simulink model "H175_Stage_01_Anode_Cathode"  (R2023a)
settings: Solver=VariableStepAuto  StartTime=0.0  StopTime=500  RelTol=1e-3
values from neighbouring files (symbols this model uses):
  anode_tube_D = 0.01    [All_Properties.mat]    (also in anode_subsystem_parameters.m; environment_parameters.m)
  D = 0.01    [All_Properties.mat]    (also in anode_subsystem_parameters.m)
  densityHydrogen = 0.0899    [All_Properties.mat]    (also in Valve_Init.m; anode_subsystem_parameters.m)
  Fischer_EMTC120K_supplier_mdot_TLU = [33.385172 57.11265182 82.35238332 173.9183787 230.2050798 50.1655574 86.1774137 122.96585 210.0188714 258.8737112 70.20710678 115.3896052 ... (25 elements, 5x5)]    [All_Properties.mat]    (also in cathode_subsystem_parameters.m = [33.385172 50.1655574 70.20710678 87.4902972 105.3161257)
  Fischer_EMTC120K_supplier_pr_TLU = [2.452176848 3.067593046 4.01020547 5.11549365 6.10066015 2.450765612 3.07166407 4.0616557 5.112468546 6.108742034 2.432340262 3.033516574 ... (25 elements, 5x5)]    [All_Properties.mat]    (also in cathode_subsystem_parameters.m = [2.452176848 2.450765612 2.432340262 2.407245766 2.37067916)
  Kv_VL6112 = 0.8    [All_Properties.mat]    (also in anode_subsystem_parameters.m)
  N2_T = [-56.55 -50 -40 -30 -20 -10 -5 -4 -3 -2 -1 0 ... (52 elements, 1x52)]    [All_Properties.mat]    (also in anode_subsystem_parameters.m = [-56.55 -50 -40 -30 -20 -10 -5 -4 -3 -2 -1 0 1 2 3 4 5 10 20; environment_parameters.m = [-56.55, -50:10:-10, -5:1:5, 10:10:350]; stack_model_harness_parameters.m = [-56.55, -50:10:-10, -5:1:5, 10:10:350])
  p_range = 0.005    [All_Properties.mat]    (also in anode_subsystem_parameters.m)
  r_max = 0.2    [All_Properties.mat]    (also in anode_subsystem_parameters.m)
  r_min = 0.0001    [All_Properties.mat]    (also in anode_subsystem_parameters.m)
  responseTimeValve = 0.013    [All_Properties.mat]    (also in anode_subsystem_parameters.m)
undefined symbols (not defined in the file or in its folder): sigbuilder_block
libraries: fl_lib x168, nesl_utility x116, SimscapeFluids_lib x8, slpidlib x5, simulink x1
(part 3 of 8)

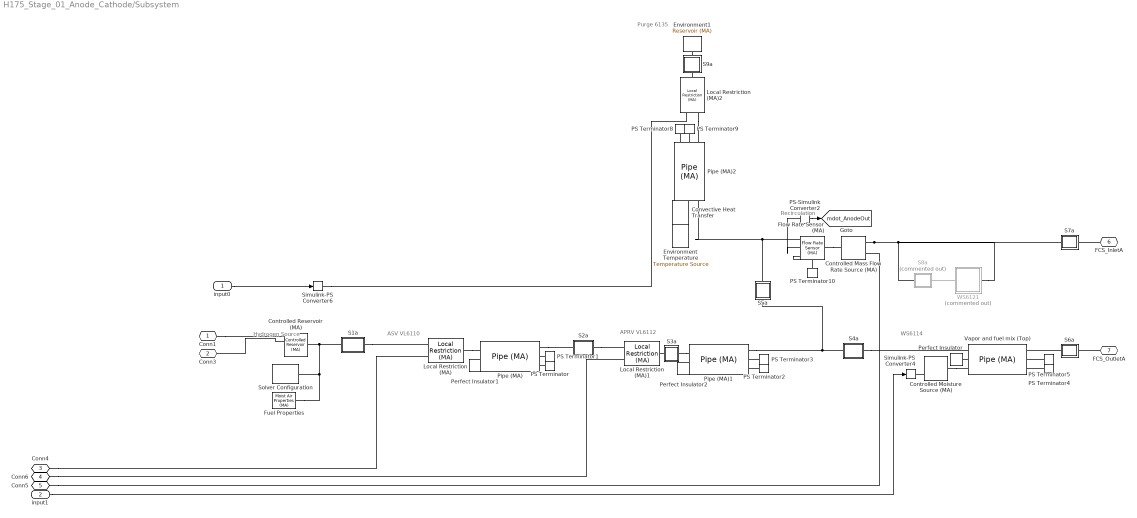
== system H175_Stage_01_Anode_Cathode/Subsystem ==
  note: Purge 6135
  note: Recirculation
  note: WS6114
  note: APRV VL6112
  note: ASV VL6110
  note: Hydrogen Source
  input0 : Inport
  input1 : Inport  Port=2
  " WS6121" : Subsystem  Tag=PublishSubsystem  Commented=on
  Controlled Mass Flow Rate Source (MA) : fl_lib/Moist Air/Sources/Controlled Mass Flow Rate Source (MA)  power_spec=foundation.enum.power_spec.isentropic  area_A=pi*anode_tube_D^2/4 m^2  area_B=pi*anode_tube_D^2/4 m^2
      settings: InternalSimscapePortConfiguration="{\"Bottom\":[],\"Left\":[{\"id\":\"A\",\"label\":\"A\",\"type\":\"foundation.moist_air.moist_air\"},{\"id\":\"M\",\"label\":\"M\",\"type\":\"input\"}],\"Right\":[{\"id\":\"B\",\"label\":\"B\",\"type\":\"foundation.moist_air.moist_air\"}],\"Top\":[]}"
  Controlled Moisture Source (MA) : fl_lib/Moist Air/Sources/Moisture & Trace Gas Sources/Controlled Moisture Source (MA)  moisture_source_spec=foundation.enum.moisture_source_spec.liquid  Phi_S_specify=off  Phi_S_priority=None  Phi_S=0 kW  Phi_S_nominal_specify=off  Phi_S_nominal_unit=kW  Phi_S_nominal_value=1  mdot_w_S_specify=off  mdot_w_S_priority=None  mdot_w_S=0 kg/s  mdot_w_S_nominal_specify=off  mdot_w_S_nominal_unit=kg/s  mdot_w_S_nominal_value=1
      settings: InternalSimscapePortConfiguration="{\"Bottom\":[],\"Left\":[{\"id\":\"S\",\"label\":\"S\",\"type\":\"foundation.moist_air.moist_air_source\"}],\"Right\":[{\"id\":\"M\",\"label\":\"M\",\"type\":\"input\"},{\"id\":\"T\",\"label\":\"T\",\"type\":\"input\"}],\"Top\":[]}"
  Controlled Reservoir (MA) : fl_lib/Moist Air/Elements/Controlled Reservoir (MA)  moisture_spec=foundation.enum.moistureSpec.RelativeHumidity  trace_gas_spec=foundation.enum.trace_gas_spec.mass_fraction  RH_ws=1  area_A=0.01 m^2  input_error_spec=foundation.enum.input_range_error.warn
      settings: InternalSimscapePortConfiguration="{\"Bottom\":[],\"Left\":[{\"id\":\"A\",\"label\":\"A\",\"type\":\"foundation.moist_air.moist_air\"}],\"Right\":[{\"id\":\"T\",\"label\":\"T\",\"type\":\"input\"},{\"id\":\"P\",\"label\":\"P\",\"type\":\"input\"},{\"id\":\"W\",\"label\":\"W\",\"type\":\"input\"},{\"id\":\"G\",\"label\":\"G\",\"type\":\"input\"}],\"Top\":[]}"
  Convective Heat Transfer : fl_lib/Thermal/Thermal Elements/Convective Heat Transfer  thermal_type=foundation.enum.constant_variable.constant  area=pi*anode_tube_D*1 m^2  heat_tr_coeff=20 W/(m^2 * K)  min_heat_tr_coeff=1e-3 W/(K*m^2)  T_specify=off  T_priority=None  T=0 K  T_nominal_specify=off  T_nominal_unit=K  T_nominal_value=1  Q_specify=off  Q_priority=None  Q=0 W  Q_nominal_specify=off  Q_nominal_unit=W  Q_nominal_value=1
  Environment Temperature : fl_lib/Thermal/Thermal Sources/Temperature Source  temperature=env_T degC
  Environment1 : fl_lib/Moist Air/Elements/Reservoir (MA)  pressure_spec=foundation.enum.pressure_spec.atmospheric  reservoir_pressure=0.101325 MPa  temperature_spec=foundation.enum.temperature_spec.atmospheric  reservoir_temperature=293.15 K  moisture_spec=foundation.enum.moistureSpec.RelativeHumidity  reservoir_RH=0.5  reservoir_x_w=0.01  reservoir_y_w=0.01  reservoir_HR=0.01  reservoir_Tw=287 K  trace_gas_spec=foundation.enum.trace_gas_spec.mass_fraction  reservoir_x_g=0.001  reservoir_y_g=0.001  RH_ws=1  area_A=0.01 m^2
  Flow Rate Sensor (MA) : fl_lib/Moist Air/Sensors/Flow Rate Sensor (MA)  mass_flow_measure=true  volumetric_flow_measure=false  volumetric_flow_conditions=foundation.enum.volumetric_flow_conditions.actual  p_std=0.101325 MPa  T_std=20 degC  RH_std=0.65  energy_flow_measure=true  vapor_flow_measure=false  gas_flow_measure=false
      settings: InternalSimscapePortConfiguration="{\"Bottom\":[{\"id\":\"PHI\",\"label\":\"φ\",\"type\":\"output\"}],\"Left\":[{\"id\":\"A\",\"label\":\"A\",\"type\":\"foundation.moist_air.moist_air\"}],\"Right\":[{\"id\":\"B\",\"label\":\"B\",\"type\":\"foundation.moist_air.moist_air\"},{\"id\":\"M\",\"label\":\"M\",\"type\":\"output\"}],\"Top\":[]}"
  Fuel Properties : fl_lib/Moist Air/Utilities/Moist Air Properties (MA)  R_a=N2_R J/kg/K  T_TLU=N2_T degC  h_a_TLU=N2_h kJ/kg  mu_a_TLU=N2_mu s*uPa  k_a_TLU=N2_k mW/m/K  p_min=1 kPa  p_max=inf MPa  T_min=min(N2_T) degC  T_max=max(N2_T) degC  properties_range_check=simscape.enum.assert.action.error  p_atm=0.101325 MPa  T_atm=20 degC  R_w=461.523 J/kg/K  p_ws_TLU=[1.71168953425982e-06; 3.93770601979424e-06; 1.28411717710344e-05; 3.80051394873809e-05; .00010323902900209; .000259873810798063; .000401741022116384; .000437454836117844; .000476040820618202; .000517704666185737; .000562664883741207; .000611212677444345; .000657088049117899; .000705987905898279; .000758082381149132; .000813549384183233; .000872574861129522; .00122818386934022; .0023392147667769; .00424668834054807; .00738442748706953; .0123512704340234; .0199458019246787; .0312006356960619; .0474147199263783; .0701823607447713; .10141797792131; .143375967241115; .198665399739302; .270259606559999; .361500961984849; .476101381081492; .618139196722055; .792053183687694; 1.0026345688121; 1.25501792086105; 1.55467186826983; 1.90739066433297; 2.31928772772542; 2.79679245576864; 3.34665187151016; 3.97593907083533; 4.69207105435535; 5.5028394740883; 6.41645928168037; 7.4416425436169; 8.58770832955728; 9.86474556030261; 11.2838558865497; 12.8575218898034; 14.6001810568052; 16.5291642526045] MPa  h_w_vap_TLU=[2836.88241275372; 2837.81392500514; 2838.63937175807; 2838.7309929628; 2838.06905313927; 2836.62597341095; 2835.60023952573; 2835.37006381376; 2835.13143158077; 2834.88429145066; 2834.62859062897; 2500.93420564316; 2498.55329907119; 2496.17495082036; 2493.79885912205; 2491.42474723191; 2489.05236104642; 2477.20875029194; 2453.54955988604; 2429.83856603313; 2406.00136954922; 2381.97406342174; 2357.69101156389; 2333.08088387814; 2308.06565480412; 2282.56034405021; 2256.47287422313; 2229.70428017508; 2202.14968030993; 2173.69998896199; 2144.24368406447; 2113.66758247452; 2081.85585110571; 2048.68725710494; 2014.03141249899; 1977.7449923284; 1939.66849592886; 1899.62342931686; 1857.40930169838; 1812.79975416601; 1765.53721731251; 1715.32525772152; 1661.81700477787; 1604.59703745016; 1543.1534616334; 1476.83692476464; 1404.80240352424; 1325.92091736114; 1238.61667822208; 1140.5102987018; 1027.62017777647; 892.733785613825] kJ/kg  h_w_TLU=[2396.55944251649; 2408.68643343608; 2427.1988031141; 2445.702165897; 2464.18429108356; 2482.62529466839; 2491.82135326629; 2493.6580151792; 2495.49372578218; 2497.32843835745; 2499.16210446923; 2500.99462758899; 2502.83092214066; 2504.6665223621; 2506.50140563013; 2508.335548891; 2510.16892865793; 2519.32352241995; 2537.56068088674; 2555.67742615292; 2573.6403223998; 2591.4109179101; 2608.9455037701; 2626.19492016262; 2643.10444358428; 2659.61377634497; 2675.58278696023; 2696.1846256545; 2716.49989553741; 2736.6235210957; 2756.61216047011; 2776.50561773853; 2796.33378922508; 2816.11979583049; 2835.88181423877; 2855.63430574511; 2875.38889327595; 2895.15500577172; 2914.94035964689; 2934.75132290228; 2954.59319330244; 2974.47041285505; 2994.38673458964; 3014.34535328009; 3034.34900867103; 3054.40006755764; 3074.50058946898; 3094.65237953784; 3114.85703128106; 3135.11596137801; 3155.43043805905; 3175.80160435813] kJ/kg  mu_w_TLU=[6.81365662228272; 7.04953750742707; 7.40970098298307; 7.76991278093907; 8.13017290129507; 8.49048134405107; 8.67065368632907; 8.70668960445667; 8.74272600580827; 8.77876289038387; 8.81480025818347; 8.85083810920707; 8.88687644345467; 8.92291526092627; 8.95895456162187; 8.99499434554147; 9.03103461268507; 9.21124319676307; 9.57169660671907; 9.93219833907507; 10.2927483938311; 10.6533467709871; 11.0139934705431; 11.3746884924991; 11.7354318368551; 12.0962235036111; 12.4570634927671; 12.8179518043231; 13.1788884382791; 13.5398733946351; 13.9009066733911; 14.2619882745471; 14.6231181981031; 14.9842964440591; 15.3455230124151; 15.7067979031711; 16.0681211163271; 16.4294926518831; 16.7909125098391; 17.1523806901951; 17.5138971929511; 17.8754620181071; 18.2370751656631; 18.5987366356191; 18.9604464279751; 19.3222045427311; 19.6840109798871; 20.0458657394431; 20.4077688213991; 20.7697202257551; 21.1317199525111; 21.4937680016671] s*uPa  k_w_TLU=[11.46288215976; 11.941997488935; 12.676358586935; 13.414208884935; 14.155548382935; 14.900377080935; 15.274099879935; 15.348949115735; 15.423833243535; 15.498752263335; 15.573706175135; 15.648694978935; 15.723718674735; 15.798777262535; 15.873870742335; 15.948999114135; 16.024162377935; 16.400502076935; 17.155798374935; 17.914583872935; 18.676858570935; 19.442622468935; 20.211875566935; 20.984617864935; 21.760849362935; 22.540570060935; 23.323779958935; 24.110479056935; 24.900667354935; 25.694344852935; 26.491511550935; 27.292167448935; 28.096312546935; 28.903946844935; 29.715070342935; 30.529683040935; 31.347784938935; 32.169376036935; 32.994456334935; 33.823025832935; 34.655084530935; 35.490632428935; 36.329669526935; 37.172195824935; 38.018211322935; 38.867716020935; 39.720709918935; 40.577193016935; 41.437165314935; 42.300626812935; 43.167577510935; 44.038017408935] mW/m/K  D_w=25 mm^2/s  trace_gas_model=foundation.enum.trace_gas_model.track_properties  R_g=H2_R J/kg/K  h_g_TLU=H2_h kJ/kg  mu_g_TLU=H2_mu s*uPa  k_g_TLU=H2_k mW/m/K  D_g=H2_D mm^2/s
      settings: AttributesFormatString=|
      | dry air --> N2
      | water vapor --> H2O
      | trace gas --> H2
  Local Restriction (MA) : fl_lib/Moist Air/Elements/Local Restriction (MA)  restriction_type=foundation.enum.restriction_type.variable  restriction_area=0.005 m^2  min_area=0.00001e-6 m^2  max_area=4.75e-6 m^2  area=0.00358 m^2  Cd=0.80  B_lam=0.999
      settings: LogSimulationData=on
  Local Restriction (MA)1 : fl_lib/Moist Air/Elements/Local Restriction (MA)  restriction_type=foundation.enum.restriction_type.variable  restriction_area=0.005 m^2  min_area=0.00001e-6 m^2  max_area=4.75e-6 m^2  area=0.00358 m^2  Cd=0.80  B_lam=0.999
      settings: LogSimulationData=on
  Local Restriction (MA)2 : fl_lib/Moist Air/Elements/Local Restriction (MA)  restriction_type=foundation.enum.restriction_type.variable  restriction_area=0.005 m^2  min_area=0.00001e-6 m^2  max_area=3.2e-6 m^2  area=0.00358 m^2  Cd=0.80  B_lam=0.999
      settings: LogSimulationData=on
  PS Terminator{,1..5,8..10} (9 alike) : fl_lib/Physical Signals/Sinks/PS Terminator
  PS-Simulink Converter2 : nesl_utility/PS-Simulink Converter  PhysicalDomain=network_engine_domain  SubClassName=ps_output  LeftPortType=input  RightPortType=output  PseudoPeriodic=off  Frequencies=[]  VectorFormat=inherit  Unit=inherit  AffineConversion=off
  Perfect Insulator : fl_lib/Thermal/Thermal Elements/Perfect Insulator  T_specify=off  T_priority=None  T=0 K  T_nominal_specify=off  T_nominal_unit=K  T_nominal_value=1
  Perfect Insulator1 : fl_lib/Thermal/Thermal Elements/Perfect Insulator  T_specify=off  T_priority=None  T=0 K  T_nominal_specify=off  T_nominal_unit=K  T_nominal_value=1
  Perfect Insulator2 : fl_lib/Thermal/Thermal Elements/Perfect Insulator  T_specify=off  T_priority=None  T=0 K  T_nominal_specify=off  T_nominal_unit=K  T_nominal_value=1
  Pipe (MA) : fl_lib/Moist Air/Elements/Pipe (MA)  length=1 m  area=pi*anode_tube_D^2/4 m^2  Dh=anode_tube_D m  length_add=0.1 m  roughness=15e-6 m  Re_lam=2000  Re_tur=4000  shape_factor=64  Nu_lam=3.66  wall_condensation=simscape.enum.onoff.off  RH_ws=1  time_constant=1e-3 s  moisture_trace_gas_source=foundation.enum.moisture_trace_gas_source.none  moisture_source_spec=foundation.enum.moisture_source_spec.vapor  moisture_mass_flow=0 kg/s  moisture_temperature_spec=foundation.enum.temperature_spec.atmospheric  moisture_temperature=293.15 K  trace_gas_mass_flow=0 kg/s  trace_gas_temperature_spec=foundation.enum.temperature_spec.atmospheric  trace_gas_temperature=293.15 K  p_I_specify=on  p_I_priority=High  p_I=env_p MPa  p_I_nominal_specify=off  p_I_nominal_unit=MPa  p_I_nominal_value=1  T_I_specify=on  T_I_priority=High  T_I=env_T degC  T_I_nominal_specify=off  T_I_nominal_unit=K  T_I_nominal_value=1  RH_I_specify=off  RH_I_priority=High  RH_I=0  RH_I_nominal_specify=off  RH_I_nominal_unit=1  RH_I_nominal_value=1  x_w_I_specify=off  x_w_I_priority=None  x_w_I=0  x_w_I_nominal_specify=off  x_w_I_nominal_unit=1  x_w_I_nominal_value=1  y_w_I_specify=off  y_w_I_priority=None  y_w_I=0  y_w_I_nominal_specify=off  y_w_I_nominal_unit=1  y_w_I_nominal_value=1  HR_I_specify=off  HR_I_priority=None  HR_I=0  HR_I_nominal_specify=off  HR_I_nominal_unit=1  HR_I_nominal_value=1  x_g_I_specify=on  x_g_I_priority=None  x_g_I=0  x_g_I_nominal_specify=off  x_g_I_nominal_unit=1  x_g_I_nominal_value=1  y_g_I_specify=on  y_g_I_priority=High  y_g_I=tank_yH2  y_g_I_nominal_specify=off  y_g_I_nominal_unit=1  y_g_I_nominal_value=1
  Pipe (MA)1 : fl_lib/Moist Air/Elements/Pipe (MA)  length=1 m  area=pi*anode_tube_D^2/4 m^2  Dh=anode_tube_D m  length_add=0.1 m  roughness=15e-6 m  Re_lam=2000  Re_tur=4000  shape_factor=64  Nu_lam=3.66  wall_condensation=simscape.enum.onoff.off  RH_ws=1  time_constant=1e-3 s  moisture_trace_gas_source=foundation.enum.moisture_trace_gas_source.none  moisture_source_spec=foundation.enum.moisture_source_spec.vapor  moisture_mass_flow=0 kg/s  moisture_temperature_spec=foundation.enum.temperature_spec.atmospheric  moisture_temperature=293.15 K  trace_gas_mass_flow=0 kg/s  trace_gas_temperature_spec=foundation.enum.temperature_spec.atmospheric  trace_gas_temperature=293.15 K  p_I_specify=on  p_I_priority=High  p_I=env_p MPa  p_I_nominal_specify=off  p_I_nominal_unit=MPa  p_I_nominal_value=1  T_I_specify=on  T_I_priority=High  T_I=env_T degC  T_I_nominal_specify=off  T_I_nominal_unit=K  T_I_nominal_value=1  RH_I_specify=off  RH_I_priority=High  RH_I=0  RH_I_nominal_specify=off  RH_I_nominal_unit=1  RH_I_nominal_value=1  x_w_I_specify=off  x_w_I_priority=None  x_w_I=0  x_w_I_nominal_specify=off  x_w_I_nominal_unit=1  x_w_I_nominal_value=1  y_w_I_specify=off  y_w_I_priority=None  y_w_I=0  y_w_I_nominal_specify=off  y_w_I_nominal_unit=1  y_w_I_nominal_value=1  HR_I_specify=off  HR_I_priority=None  HR_I=0  HR_I_nominal_specify=off  HR_I_nominal_unit=1  HR_I_nominal_value=1  x_g_I_specify=on  x_g_I_priority=None  x_g_I=0  x_g_I_nominal_specify=off  x_g_I_nominal_unit=1  x_g_I_nominal_value=1  y_g_I_specify=on  y_g_I_priority=High  y_g_I=tank_yH2  y_g_I_nominal_specify=off  y_g_I_nominal_unit=1  y_g_I_nominal_value=1
  Pipe (MA)2 : fl_lib/Moist Air/Elements/Pipe (MA)  length=1 m  area=pi*anode_tube_D^2/4 m^2  Dh=anode_tube_D m  length_add=0.1 m  roughness=15e-6 m  Re_lam=2000  Re_tur=4000  shape_factor=64  Nu_lam=3.66  wall_condensation=simscape.enum.onoff.off  RH_ws=1  time_constant=1e-3 s  moisture_trace_gas_source=foundation.enum.moisture_trace_gas_source.none  moisture_source_spec=foundation.enum.moisture_source_spec.vapor  moisture_mass_flow=0 kg/s  moisture_temperature_spec=foundation.enum.temperature_spec.atmospheric  moisture_temperature=293.15 K  trace_gas_mass_flow=0 kg/s  trace_gas_temperature_spec=foundation.enum.temperature_spec.atmospheric  trace_gas_temperature=293.15 K  p_I_specify=on  p_I_priority=High  p_I=env_p MPa  p_I_nominal_specify=off  p_I_nominal_unit=MPa  p_I_nominal_value=1  T_I_specify=on  T_I_priority=High  T_I=env_T degC  T_I_nominal_specify=off  T_I_nominal_unit=K  T_I_nominal_value=1  RH_I_specify=off  RH_I_priority=High  RH_I=0  RH_I_nominal_specify=off  RH_I_nominal_unit=1  RH_I_nominal_value=1  x_w_I_specify=off  x_w_I_priority=None  x_w_I=0  x_w_I_nominal_specify=off  x_w_I_nominal_unit=1  x_w_I_nominal_value=1  y_w_I_specify=off  y_w_I_priority=None  y_w_I=0  y_w_I_nominal_specify=off  y_w_I_nominal_unit=1  y_w_I_nominal_value=1  HR_I_specify=off  HR_I_priority=None  HR_I=0  HR_I_nominal_specify=off  HR_I_nominal_unit=1  HR_I_nominal_value=1  x_g_I_specify=on  x_g_I_priority=None  x_g_I=0  x_g_I_nominal_specify=off  x_g_I_nominal_unit=1  x_g_I_nominal_value=1  y_g_I_specify=on  y_g_I_priority=High  y_g_I=tank_yH2  y_g_I_nominal_specify=off  y_g_I_nominal_unit=1  y_g_I_nominal_value=1
  S1a : Subsystem
  S2a : Subsystem
  S3a : Subsystem
  S4a : Subsystem
  S5a : Subsystem
  S6a : Subsystem
  S7a : Subsystem  Tag=PublishSubsystem
  S8a : Subsystem  Tag=PublishSubsystem  Commented=on
  S9a : Subsystem
  Simulink-PS Converter4 : nesl_utility/Simulink-PS Converter  PhysicalDomain=network_engine_domain  SubClassName=ps_input  LeftPortType=input  RightPortType=output  PseudoPeriodic=off  Frequencies=[]  NoiseDistribution=none  NoiseParameters=[]  Unit=1  AffineConversion=off  FilteringAndDerivatives=provide  SimscapeFilterOrder=1  InputFilterTimeConstant=0.001  UdotUserProvided=0
  Simulink-PS Converter6 : nesl_utility/Simulink-PS Converter  PhysicalDomain=network_engine_domain  SubClassName=ps_input  LeftPortType=input  RightPortType=output  PseudoPeriodic=off  Frequencies=[]  NoiseDistribution=none  NoiseParameters=[]  Unit=1  AffineConversion=off  FilteringAndDerivatives=provide  SimscapeFilterOrder=1  InputFilterTimeConstant=0.001  UdotUserProvided=0
  Solver Configuration : nesl_utility/Solver Configuration  PhysicalDomain=network_engine_domain  SubClassName=solver  LeftPortType=input  RightPortType=generic  Tones=[]  Harmonics=[]  SimulateNoise=off  Profile=off  UseLocalSampling=off  EnableSwitchedLinearOptims=on  FrequencyDomain=off  UseCCode=off  RelTol=0.001  AbsTol=0.001  MinStep=1e-09  ToWorkspace=off  RevertToSquareIcSolve=off  NumHomotopyIterations=100  PhasorMode=off  PhasorModeNumHarmonics=1  ConsistencySolver=NEWTON_XTOL_AFTER_FTOL  IndexReductionMethod=DerivativeReplacement  DoDC=off  ResidualTolerance=1e-09  ConsistencyTolSource=GLOBAL  ConsistencyAbsTol=0.001  ConsistencyRelTol=0.001  ConsistencyTolFactor=0.001  UseLocalSolver=off  LocalSolverChoice=NE_BACKWARD_EULER_ADVANCER  ResolveIndetEquations=on  FunctionEvalNumThread=1  LocalSolverSampleTime=0.001  DoFixedCost=off  MaxNonlinIter=3  MaxModeIter=2  ComputeImpulses=off  ImpulseIterations=2  LinearAlgebra=auto  LinearAlgebraNumThread=0  EquationFormulation=NE_TIME_EF  DelaysMemoryBudget=1024  AutomaticFiltering=on  FilteringTimeConstant=0.001  PartitionStorageMethod=AS_NEEDED  PartitionMemoryBudget=1024  PartitionMethod=ROBUST
  Vapor and fuel mix (Top) : fl_lib/Moist Air/Elements/Pipe (MA)  length=0.25 m  area=pi*0.05^2/4 m^2  Dh=0.05 m  length_add=0.1 m  roughness=15e-6 m  Re_lam=2000  Re_tur=4000  shape_factor=64  Nu_lam=3.66  wall_condensation=simscape.enum.onoff.off  RH_ws=1  time_constant=1e-3 s  moisture_trace_gas_source=foundation.enum.moisture_trace_gas_source.controlled  moisture_source_spec=foundation.enum.moisture_source_spec.vapor  moisture_mass_flow=0 kg/s  moisture_temperature_spec=foundation.enum.temperature_spec.atmospheric  moisture_temperature=293.15 K  trace_gas_mass_flow=0 kg/s  trace_gas_temperature_spec=foundation.enum.temperature_spec.atmospheric  trace_gas_temperature=293.15 K  p_I_specify=on  p_I_priority=High  p_I=env_p MPa  p_I_nominal_specify=off  p_I_nominal_unit=MPa  p_I_nominal_value=1  T_I_specify=on  T_I_priority=High  T_I=env_T degC  T_I_nominal_specify=off  T_I_nominal_unit=K  T_I_nominal_value=1  RH_I_specify=off  RH_I_priority=High  RH_I=0  RH_I_nominal_specify=off  RH_I_nominal_unit=1  RH_I_nominal_value=1  x_w_I_specify=off  x_w_I_priority=None  x_w_I=0  x_w_I_nominal_specify=off  x_w_I_nominal_unit=1  x_w_I_nominal_value=1  y_w_I_specify=off  y_w_I_priority=None  y_w_I=0  y_w_I_nominal_specify=off  y_w_I_nominal_unit=1  y_w_I_nominal_value=1  HR_I_specify=off  HR_I_priority=None  HR_I=0  HR_I_nominal_specify=off  HR_I_nominal_unit=1  HR_I_nominal_value=1  x_g_I_specify=on  x_g_I_priority=None  x_g_I=0  x_g_I_nominal_specify=off  x_g_I_nominal_unit=1  x_g_I_nominal_value=1  y_g_I_specify=on  y_g_I_priority=High  y_g_I=tank_yH2  y_g_I_nominal_specify=off  y_g_I_nominal_unit=1  y_g_I_nominal_value=1
      settings: InternalSimscapePortConfiguration="{\"Bottom\":[],\"Left\":[{\"id\":\"A\",\"label\":\"A\",\"type\":\"foundation.moist_air.moist_air\"},{\"id\":\"H\",\"label\":\"H\",\"type\":\"foundation.thermal.thermal\"},{\"id\":\"S\",\"label\":\"S\",\"type\":\"foundation.moist_air.moist_air_source\"}],\"Right\":[{\"id\":\"B\",\"label\":\"B\",\"type\":\"foundation.moist_air.moist_air\"},{\"id\":\"W\",\"label\":\"W\",\"type\":\"output\"},{\"id\":\"F\",\"label\":\"F\",\"type\":\"output\"}],\"Top\":[]}"
  Conn1 : PMIOPort  Side=Left
  Conn3 : PMIOPort  Port=2  Side=Left
  Conn4 : PMIOPort  Port=3  Side=Left
  Conn6 : PMIOPort  Port=4  Side=Left
  Conn5 : PMIOPort  Port=5  Side=Left
  FCS_InletA : PMIOPort  Port=6  Side=Right
  FCS_OutletA : PMIOPort  Port=7  Side=Right
  tag scope: mdot_AnodeOut=global
  wires:
  input1/1 -> Simulink-PS Converter4/1
  PS-Simulink Converter2/1 -> [mdot_AnodeOut]
  input0/1 -> Simulink-PS Converter6/1
  connections:
  Simulink-PS Converter4/RConn1 -- Controlled Moisture Source (MA)/RConn1
  Controlled Moisture Source (MA)/LConn1 -- Vapor and fuel mix (Top)/LConn3
  PS Terminator10/LConn1 -- Flow Rate Sensor (MA)/RConn3
  S4a/RConn1 -- Vapor and fuel mix (Top)/LConn1
  PS Terminator2/LConn1 -- Pipe (MA)1/RConn3
  Controlled Mass Flow Rate Source (MA)/LConn1 -- " WS6121"/LConn1 -- S7a/LConn1 -- S8a/LConn1
  Controlled Reservoir (MA)/RConn2 -- Conn3/RConn1
  Perfect Insulator/LConn1 -- Vapor and fuel mix (Top)/LConn2
  PS-Simulink Converter2/LConn1 -- Flow Rate Sensor (MA)/RConn2
  PS Terminator3/LConn1 -- Pipe (MA)1/RConn2
  Pipe (MA)/RConn1 -- S2a/LConn1
  S3a/RConn1 -- Pipe (MA)1/LConn1
  Pipe (MA)2/RConn2 -- PS Terminator9/LConn1
  Pipe (MA)1/RConn1 -- S4a/LConn1 -- S5a/LConn1
  PS Terminator5/LConn1 -- Vapor and fuel mix (Top)/RConn2
  S6a/LConn1 -- Vapor and fuel mix (Top)/RConn1
  Fuel Properties/RConn1 -- S1a/LConn1 -- Controlled Reservoir (MA)/LConn1 -- Solver Configuration/RConn1
  Local Restriction (MA)/RConn1 -- Pipe (MA)/LConn1
  S1a/RConn1 -- Local Restriction (MA)/LConn1
  Flow Rate Sensor (MA)/RConn1 -- Pipe (MA)2/LConn1 -- S5a/RConn1
  Pipe (MA)2/RConn3 -- PS Terminator8/LConn1
  PS Terminator1/LConn1 -- Pipe (MA)/RConn2
  Environment Temperature/LConn1 -- Convective Heat Transfer/RConn1
  Conn5/RConn1 -- Controlled Mass Flow Rate Source (MA)/LConn2
  Local Restriction (MA)2/LConn1 -- Pipe (MA)2/RConn1
  Pipe (MA)/LConn2 -- Perfect Insulator1/LConn1
  PS Terminator/LConn1 -- Pipe (MA)/RConn3
  Conn1/RConn1 -- Controlled Reservoir (MA)/RConn1
  Flow Rate Sensor (MA)/LConn1 -- Controlled Mass Flow Rate Source (MA)/RConn1
  Local Restriction (MA)1/RConn1 -- S3a/LConn1
  Convective Heat Transfer/LConn1 -- Pipe (MA)2/LConn2
  Conn6/RConn1 -- Local Restriction (MA)1/LConn2
  PS Terminator4/LConn1 -- Vapor and fuel mix (Top)/RConn3
  Perfect Insulator2/LConn1 -- Pipe (MA)1/LConn2
  S2a/RConn1 -- Local Restriction (MA)1/LConn1
  Simulink-PS Converter6/RConn1 -- Local Restriction (MA)2/LConn2
  Conn4/RConn1 -- Local Restriction (MA)/LConn2
  S9a/RConn1 -- Environment1/LConn1
  Local Restriction (MA)2/RConn1 -- S9a/LConn1
  " WS6121"/RConn1 -- S8a/RConn1
  FCS_InletA/RConn1 -- S7a/RConn1
  FCS_OutletA/RConn1 -- S6a/RConn1

== system H175_Stage_01_Anode_Cathode/System_Measurements ==
  Gain : Gain  Gain=1e-3
  Mux : Mux  Inputs=2
  Product : Product
  i : Outport
  v : Outport  Port=2
  P : Outport  Port=3
  T : Outport  Port=4
  wires:
  [v_stack] -> Product/2, v/1
  [i_stack] -> Product/1, i/1
  [T_stack] -> T/1
  [Q_stack] -> Mux/2
  Product/1 -> Gain/1
  Mux/1 -> P/1
  Gain/1 -> Mux/1

== system H175_Stage_01_Anode_Cathode/Anode Controller/APRV_VL6112 Valve_Control ==
  note: Valve Lift Command Controller calculates valvelift signal for an
      | ideal controller, to reach desired vave outlet pressure, assuming
      | a linear relation between valve lift and Kvs.
      | (funcionality validated 09.05.2023)
  Desired Control Outlet Pressure [bar] : Inport
  Control Outlet Mass Flow Rate [g/s] : Inport  Port=2
  Display : Display
  Gain4 : Gain  Gain=1e-5
  Gain5 : Gain  Gain=1000
  Kv [m^3/h] : Constant  Value=Kv_VL6112
  Saturation : Saturate  UpperLimit=1  LowerLimit=0
  Scope : Scope  NumInputPorts=2
  Simulink-PS Converter3 : nesl_utility/Simulink-PS Converter  PhysicalDomain=network_engine_domain  SubClassName=ps_input  LeftPortType=input  RightPortType=output  PseudoPeriodic=off  Frequencies=[]  NoiseDistribution=none  NoiseParameters=[]  Unit=m^2  AffineConversion=off  FilteringAndDerivatives=provide  SimscapeFilterOrder=1  InputFilterTimeConstant=0.001  UdotUserProvided=0
  Standard Density [kg/(m^3)] : Constant  Value=densityHydrogen
  Valve Lift Command Control : MATLAB Function  TreatAsAtomicUnit=on
  Valve Response [-] : TransferFcn  Numerator=[4.75e-6]  Denominator=[responseTimeValve/3 1]
  output : PMIOPort  Side=Right
  wires:
  [S2a_Pres] -> Gain4/1
  Valve Response [-]/1 -> Simulink-PS Converter3/1  "valve_opening"
  Gain5/1 -> Valve Response [-]/1
  Valve Lift Command Control/2(W) -> Display/1
  Saturation/1 -> Gain5/1, Scope/2  "lift_signal_command"
  Valve Lift Command Control/1(lift_signal) -> Saturation/1
  Standard Density [kg/(m^3)]/1 -> Valve Lift Command Control/6(rho_std)
  Kv [m^3/h]/1 -> Valve Lift Command Control/5(Kvs)
  [S2a_Temp] -> Valve Lift Command Control/4(T1)  "T_valve_in"
  Control Outlet Mass Flow Rate [g/s]/1 -> Valve Lift Command Control/1(m_dot), Scope/1  "m_dot_valve"
  Gain4/1 -> Valve Lift Command Control/2(p1)  "p_valve_in"
  Desired Control Outlet Pressure [bar]/1 -> Valve Lift Command Control/3(p2)  "p_valve_out_desired"
  connections:
  Simulink-PS Converter3/RConn1 -- output/RConn1

== system H175_Stage_01_Anode_Cathode/Anode Controller/ASVValve_Control ==
  PS Add : fl_lib/Physical Signals/Functions/PS Add
  PS Constant : fl_lib/Physical Signals/Sources/PS Constant  constant=r_max^2
  PS Gain : fl_lib/Physical Signals/Functions/PS Gain  gain=(r_min^2 - r_max^2)/p_range
  PS Gain1 : fl_lib/Physical Signals/Functions/PS Gain  gain=pi*D^2/4 m^2
  PS Subtract : fl_lib/Physical Signals/Functions/PS Subtract
  Pa to MPa : fl_lib/Physical Signals/Functions/PS Gain  gain=.000001
  Simulink-PS Converter : nesl_utility/Simulink-PS Converter  PhysicalDomain=network_engine_domain  SubClassName=ps_input  LeftPortType=input  RightPortType=output  PseudoPeriodic=off  Frequencies=[]  NoiseDistribution=none  NoiseParameters=[]  Unit=1  AffineConversion=off  FilteringAndDerivatives=provide  SimscapeFilterOrder=1  InputFilterTimeConstant=0.001  UdotUserProvided=0
  Conn3 : PMIOPort  Side=Left
  Conn1 : PMIOPort  Port=2  Side=Right
  wires:
  [S2a_Pres] -> Simulink-PS Converter/1
  connections:
  PS Gain1/RConn1 -- Conn1/RConn1
  PS Add/RConn1 -- PS Gain1/LConn1
  PS Constant/RConn1 -- PS Add/LConn1
  PS Subtract/LConn2 -- Conn3/RConn1
  PS Gain/LConn1 -- Pa to MPa/RConn1
  PS Add/LConn2 -- PS Gain/RConn1
  Simulink-PS Converter/RConn1 -- PS Subtract/LConn1
  Pa to MPa/LConn1 -- PS Subtract/RConn1

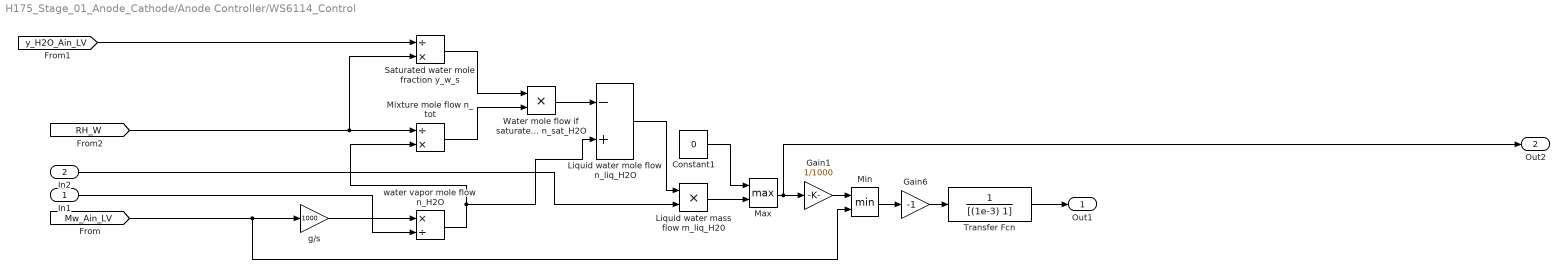
== system H175_Stage_01_Anode_Cathode/Anode Controller/WS6114_Control ==
  In1 : Inport
  In2 : Inport  Port=2
  Constant1 : Constant  Value=0
  Gain1 : Gain  Gain=1/1000
  Gain6 : Gain  Gain=-1
  Liquid water mass flow m_liq_H20 : Product
  Liquid water mole flow n_liq_H2O : Sum  Inputs=-+
  Max : MinMax  Function=max  Inputs=2
  Min : MinMax  Inputs=2
  Mixture mole flow n_tot : Product  Inputs=/*
  Saturated water mole fraction y_w_s : Product  Inputs=/*
  Transfer Fcn : TransferFcn  Denominator=[(1e-3) 1]
  Water mole flow if saturated n_sat_H2O : Product
  g/s : Gain  Gain=1000
  water vapor mole flow n_H2O : Product  Inputs=*/
  Out1 : Outport
  Out2 : Outport  Port=2
  wires:
  Max/1 -> Out2/1, Gain1/1
  [Mw_Ain_LV] -> Min/2, g/s/1
  water vapor mole flow n_H2O/1 -> Mixture mole flow n_tot/2, Liquid water mole flow n_liq_H2O/2
  Min/1 -> Gain6/1
  Constant1/1 -> Max/1
  In1/1 -> water vapor mole flow n_H2O/2
  g/s/1 -> water vapor mole flow n_H2O/1
  Liquid water mole flow n_liq_H2O/1 -> Liquid water mass flow m_liq_H20/1
  In2/1 -> Liquid water mass flow m_liq_H20/2
  Gain1/1 -> Min/1
  Gain6/1 -> Transfer Fcn/1
  Mixture mole flow n_tot/1 -> Water mole flow if saturated n_sat_H2O/2
  Liquid water mass flow m_liq_H20/1 -> Max/2
  Water mole flow if saturated n_sat_H2O/1 -> Liquid water mole flow n_liq_H2O/1
  [RH_W] -> Mixture mole flow n_tot/1, Saturated water mole fraction y_w_s/2
  Transfer Fcn/1 -> Out1/1
  [y_H2O_Ain_LV] -> Saturated water mole fraction y_w_s/1
  Saturated water mole fraction y_w_s/1 -> Water mole flow if saturated n_sat_H2O/1

== system H175_Stage_01_Anode_Cathode/Anode Controller/compressor map ==
  Constant4 : Constant  Value=0.0899
  Constant5 : Constant  Value=2
  Display : Display
  PS Gain : fl_lib/Physical Signals/Functions/PS Gain  gain=1/3600
  PS Lookup Table (2D) : fl_lib/Physical Signals/Lookup Tables/PS Lookup Table (2D)  x1=comp6122_p_out  x2=comp6122_rpm  f=comp6122_V_dot  interp_method=simscape.enum.interpolation.linear  extrap_method=simscape.enum.extrapolation.linear
  PS Product : fl_lib/Physical Signals/Functions/PS Product
  PS Product1 : fl_lib/Physical Signals/Functions/PS Product
  PS-Simulink Converter1 : nesl_utility/PS-Simulink Converter  PhysicalDomain=network_engine_domain  SubClassName=ps_output  LeftPortType=input  RightPortType=output  PseudoPeriodic=off  Frequencies=[]  VectorFormat=inherit  Unit=inherit  AffineConversion=off
  Simulink-PS Converter5 : nesl_utility/Simulink-PS Converter  PhysicalDomain=network_engine_domain  SubClassName=ps_input  LeftPortType=input  RightPortType=output  PseudoPeriodic=off  Frequencies=[]  NoiseDistribution=none  NoiseParameters=[]  Unit=1  AffineConversion=on  FilteringAndDerivatives=provide  SimscapeFilterOrder=1  InputFilterTimeConstant=0.001  UdotUserProvided=0
  Simulink-PS Converter6 : nesl_utility/Simulink-PS Converter  PhysicalDomain=network_engine_domain  SubClassName=ps_input  LeftPortType=input  RightPortType=output  PseudoPeriodic=off  Frequencies=[]  NoiseDistribution=none  NoiseParameters=[]  Unit=1  AffineConversion=on  FilteringAndDerivatives=provide  SimscapeFilterOrder=1  InputFilterTimeConstant=0.001  UdotUserProvided=0
  p : PMIOPort  Side=Left
  cmd : PMIOPort  Port=2  Side=Right
  rpm : PMIOPort  Port=3  Side=Left
  wires:
  Constant4/1 -> Simulink-PS Converter5/1
  Constant5/1 -> Simulink-PS Converter6/1
  PS-Simulink Converter1/1 -> Display/1
  connections:
  Simulink-PS Converter5/RConn1 -- PS Product/LConn2
  PS Lookup Table (2D)/RConn1 -- PS Gain/LConn1 -- PS-Simulink Converter1/LConn1
  PS Product/RConn1 -- PS Product1/LConn1
  PS Product/LConn1 -- PS Gain/RConn1
  PS Lookup Table (2D)/LConn2 -- rpm/RConn1
  Simulink-PS Converter6/RConn1 -- PS Product1/LConn2
  PS Product1/RConn1 -- cmd/RConn1
  p/RConn1 -- PS Lookup Table (2D)/LConn1

== system H175_Stage_01_Anode_Cathode/Cathode_Plant_Sensors/EAC_Theo_Power ==
  <mFlow_S1> : Inport
  <aPres_S1> : Inport  Port=2
  <aPres_S2> : Inport  Port=3
  <aTemp_S1> : Inport  Port=4
  Cp : Constant  Value=1004
  Divide : Product  Inputs=*/
  MATLAB Function : MATLAB Function  TreatAsAtomicUnit=on
  Product : Product  Inputs=4
  y-exp : Constant  Value=(1.33-1)/1.33
  Out1 : Outport
  wires:
  Cp/1 -> Product/1
  <aTemp_S1>/1 -> Product/2
  <aPres_S1>/1 -> Divide/2
  Product/1 -> Out1/1
  <aPres_S2>/1 -> Divide/1
  MATLAB Function/1(y) -> Product/4
  y-exp/1 -> MATLAB Function/2(data)
  Divide/1 -> MATLAB Function/1(u)
  <mFlow_S1>/1 -> Product/3

== system H175_Stage_01_Anode_Cathode/Cathode_Plant_Sensors/EAT_Theo_Power ==
  <mFlow_S1> : Inport
  <aPres_S6> : Inport  Port=2
  <aTemp_S6> : Inport  Port=3
  <aPres_S7> : Inport  Port=4
  Cp : Constant  Value=1150
  Divide : Product  Inputs=*/
  Gain : Gain  Gain=-1
  MATLAB Function : MATLAB Function  TreatAsAtomicUnit=on
  Product : Product  Inputs=4
  y-exp : Constant  Value=(1.33-1)/1.33
  Out1 : Outport
  wires:
  y-exp/1 -> MATLAB Function/2(data)
  <aPres_S7>/1 -> Divide/1
  Cp/1 -> Product/4
  Divide/1 -> MATLAB Function/1(u)
  Product/1 -> Gain/1
  <mFlow_S1>/1 -> Product/2
  MATLAB Function/1(y) -> Product/1
  <aTemp_S6>/1 -> Product/3
  <aPres_S6>/1 -> Divide/2
  Gain/1 -> Out1/1

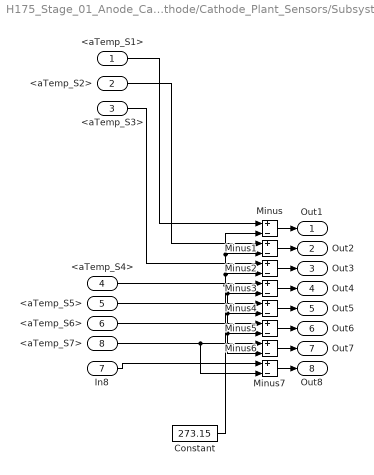
== system H175_Stage_01_Anode_Cathode/Cathode_Plant_Sensors/Subsystem ==
  <aTemp_S1> : Inport
  <aTemp_S2> : Inport  Port=2
  <aTemp_S3> : Inport  Port=3
  <aTemp_S4> : Inport  Port=4
  <aTemp_S5> : Inport  Port=5
  <aTemp_S6> : Inport  Port=6
  In8 : Inport  Port=7
  <aTemp_S7> : Inport  Port=8
  Constant : Constant  Value=273.15
  Minus{,1..7} (8 alike) : Sum  Inputs=+-
  Out1 : Outport
  Out2 : Outport  Port=2
  Out3 : Outport  Port=3
  Out4 : Outport  Port=4
  Out5 : Outport  Port=5
  Out6 : Outport  Port=6
  Out7 : Outport  Port=7
  Out8 : Outport  Port=8
  wires:
  Minus4/1 -> Out5/1
  Constant/1 -> Minus6/2, Minus5/2, Minus4/2, Minus3/2, Minus2/2, Minus1/2, Minus/2
  Minus2/1 -> Out3/1
  <aTemp_S7>/1 -> Minus7/2, Minus6/1
  <aTemp_S4>/1 -> Minus3/1
  <aTemp_S1>/1 -> Minus/1
  Minus5/1 -> Out6/1
  Minus6/1 -> Out7/1
  <aTemp_S3>/1 -> Minus2/1
  Minus/1 -> Out1/1
  <aTemp_S5>/1 -> Minus4/1
  Minus3/1 -> Out4/1
  Minus1/1 -> Out2/1
  <aTemp_S6>/1 -> Minus5/1
  <aTemp_S2>/1 -> Minus1/1
  In8/1 -> Minus7/1
  Minus7/1 -> Out8/1

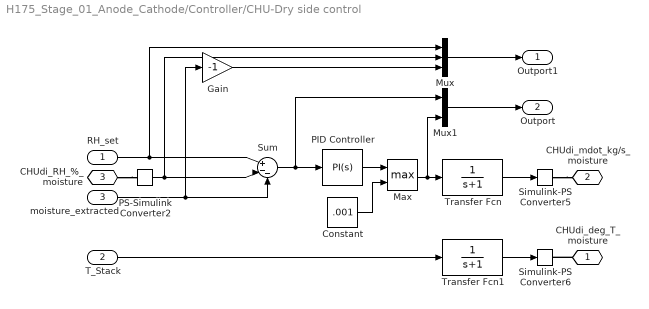
== system H175_Stage_01_Anode_Cathode/Controller/CHU-Dry side control ==
  RH_set : Inport
  T_Stack : Inport  Port=2
  moisture_extracted : Inport  Port=3
  Constant : Constant  Value=.001
  Gain : Gain  Gain=-1
  Max : MinMax  Function=max  Inputs=2
  Mux : Mux  Inputs=3
  Mux1 : Mux  Inputs=2
  PID Controller : slpidlib/PID Controller  Controller=PI  Form=Parallel  TimeDomain=Continuous-time  UseExternalTs=off  SampleTime=-1  IntegratorMethod=Forward Euler  FilterMethod=Forward Euler  ControllerParametersSource=internal  P=1  I=1  UseKiTs=off  D=0  N=100  UseFilter=on  TunerSelectOption=Transfer Function Based (PID Tuner App)  InitialConditionSource=internal  InitialConditionForIntegrator=0  InitialConditionForFilter=0  DifferentiatorICPrevScaledInput=0  ExternalReset=none  TrackingMode=off  Kt=1  LimitOutput=off  SatLimitsSource=internal  UpperSaturationLimit=inf  LowerSaturationLimit=-inf  LinearizeAsGain=on  AntiWindupMode=none  Kb=1  LimitIntegrator=off  UpperIntegratorSaturationLimit=inf  LowerIntegratorSaturationLimit=-inf  POutMin=[]  POutMax=[]  IOutMin=[]  IOutMax=[]  DOutMin=[]  DOutMax=[]  NOutMin=[]  NOutMax=[]  SumOutMin=[]  SumOutMax=[]  SaturationOutMin=[]  SaturationOutMax=[]  PParamMin=[]  PParamMax=[]  IParamMin=[]  IParamMax=[]  DParamMin=[]  DParamMax=[]  NParamMin=[]  NParamMax=[]  KbParamMin=[]  KbParamMax=[]  KtParamMin=[]  KtParamMax=[]  KbOutMin=[]  KbOutMax=[]  KtOutMin=[]  KtOutMax=[]  IntegratorOutMin=[]  IntegratorOutMax=[]  FilterOutMin=[]  FilterOutMax=[]  SumI1OutMin=[]  SumI1OutMax=[]  SumI2OutMin=[]  SumI2OutMax=[]  SumI3OutMin=[]  SumI3OutMax=[]  SumI4OutMin=[]  SumI4OutMax=[]  SumDOutMin=[]  SumDOutMax=[]  DifferentiatorOutMin=[]  DifferentiatorOutMax=[]  FilterDiffOutCoefMin=[]  FilterDiffOutCoefMax=[]  ReciprocalOutMin=[]  ReciprocalOutMax=[]  SumDenOutMin=[]  SumDenOutMax=[]  SumNumOutMin=[]  SumNumOutMax=[]  DivideOutMin=[]  DivideOutMax=[]  UdiffTsProdOutMin=[]  UdiffTsProdOutMax=[]  NTsProdOutMin=[]  NTsProdOutMax=[]  UintegralTsProdOutMin=[]  UintegralTsProdOutMax=[]  UngainTsProdOutMin=[]  UngainTsProdOutMax=[]  ClampingZeroOutDataTypeStr=Inherit: Inherit via back propagation  ClampingZeroOutMin=[]  ClampingZeroOutMax=[]  FilterDenConstantOutDataTypeStr=Inherit: Inherit via back propagation  FilterDenConstantOutMin=[]  FilterDenConstantOutMax=[]  PCopyOutDataTypeStr=Inherit: Inherit via back propagation  PCopyOutMin=[]  PCopyOutMax=[]  NCopyOutDataTypeStr=Inherit: Inherit via back propagation  NCopyOutMin=[]  NCopyOutMax=[]  IntegratorContinuousStateAttributes=''  IntegratorStateMustResolveToSignalObject=off  IntegratorRTWStateStorageClass=Auto  FilterContinuousStateAttributes=''  FilterStateMustResolveToSignalObject=off  FilterRTWStateStorageClass=Auto  ParallelPVariant=InternalParameters  IdealPVariant=Disabled  IVariant=InternalParameters  DVariant=Disabled  IntegratorVariant=Continuous  SatVariant=Disabled  AWVariant=Passthrough  PCopyVariant=Disabled  TRVariant=Disabled  FdbkBlocksVariant=Forward  IdealPFdbkVariant=Disabled  SatFdbkVariant=Disabled  DerivativeFilterVariant=Disabled  NVariant=Disabled  NCopyVariant=Disabled_SignalSpec  FilterICVariant=Disabled  IntegratorICVariant=InternalICs  ExternalResetVariant=Disabled  TRSumVariant=Passthrough  SumFdbkVariant=Disabled  SumVariant=Sum_PI  TsampFilterVariant=InternalTs  TsampNgainVariant=Passthrough  TsampIntegralVariant=Disabled_SignalSpec  ExternalSaturationOutDataTypeStr=Inherit: Same as second input
  PS-Simulink Converter2 : nesl_utility/PS-Simulink Converter  PhysicalDomain=network_engine_domain  SubClassName=ps_output  LeftPortType=input  RightPortType=output  PseudoPeriodic=off  Frequencies=[]  VectorFormat=1-D array  Unit=1  AffineConversion=off
  Simulink-PS Converter5 : nesl_utility/Simulink-PS Converter  PhysicalDomain=network_engine_domain  SubClassName=ps_input  LeftPortType=input  RightPortType=output  PseudoPeriodic=off  Frequencies=[]  NoiseDistribution=none  NoiseParameters=[]  Unit=kg/s  AffineConversion=off  FilteringAndDerivatives=provide  SimscapeFilterOrder=1  InputFilterTimeConstant=0.001  UdotUserProvided=0
  Simulink-PS Converter6 : nesl_utility/Simulink-PS Converter  PhysicalDomain=network_engine_domain  SubClassName=ps_input  LeftPortType=input  RightPortType=output  PseudoPeriodic=off  Frequencies=[]  NoiseDistribution=none  NoiseParameters=[]  Unit=degC  AffineConversion=on  FilteringAndDerivatives=provide  SimscapeFilterOrder=1  InputFilterTimeConstant=0.001  UdotUserProvided=0
  Sum : Sum  Inputs=|+--
  Transfer Fcn : TransferFcn  Denominator=[1 1]
  Transfer Fcn1 : TransferFcn  Denominator=[1 1]
  CHUdi_deg_T_moisture : PMIOPort  Side=Right
  CHUdi_mdot_kg/s_moisture : PMIOPort  Port=2  Side=Right
  CHUdi_RH_%_moisture : PMIOPort  Port=3  Side=Right
  Outport1 : Outport
  Outport : Outport  Port=2
  wires:
  Transfer Fcn/1 -> Simulink-PS Converter5/1
  T_Stack/1 -> Transfer Fcn1/1
  Transfer Fcn1/1 -> Simulink-PS Converter6/1
  Max/1 -> Mux1/2, Transfer Fcn/1
  Constant/1 -> Max/2
  moisture_extracted/1 -> Gain/1, Sum/3
  PID Controller/1 -> Max/1
  PS-Simulink Converter2/1 -> Mux/2, Sum/2
  Sum/1 -> Mux1/1, PID Controller/1
  RH_set/1 -> Mux/1, Sum/1
  Mux/1 -> Outport1/1
  Mux1/1 -> Outport/1
  Gain/1 -> Mux/3
  connections:
  Simulink-PS Converter5/RConn1 -- CHUdi_mdot_kg/s_moisture/RConn1
  CHUdi_deg_T_moisture/RConn1 -- Simulink-PS Converter6/RConn1
  CHUdi_RH_%_moisture/RConn1 -- PS-Simulink Converter2/LConn1

== system H175_Stage_01_Anode_Cathode/Controller/CHU-wet side control ==
  T_Stack : Inport
  RH_set : Inport  Port=2
  Mux : Mux  Inputs=2
  Mux1 : Mux  Inputs=2
  PS-Simulink Converter : nesl_utility/PS-Simulink Converter  PhysicalDomain=network_engine_domain  SubClassName=ps_output  LeftPortType=input  RightPortType=output  PseudoPeriodic=off  Frequencies=[]  VectorFormat=1-D array  Unit=1  AffineConversion=off
  Saturation : Saturate  UpperLimit=inf  LowerLimit=-.2  ZeroCross=off
  Simulink-PS Converter : nesl_utility/Simulink-PS Converter  PhysicalDomain=network_engine_domain  SubClassName=ps_input  LeftPortType=input  RightPortType=output  PseudoPeriodic=off  Frequencies=[]  NoiseDistribution=none  NoiseParameters=[]  Unit=kg/s  AffineConversion=off  FilteringAndDerivatives=provide  SimscapeFilterOrder=1  InputFilterTimeConstant=0.001  UdotUserProvided=0
  Simulink-PS Converter2 : nesl_utility/Simulink-PS Converter  PhysicalDomain=network_engine_domain  SubClassName=ps_input  LeftPortType=input  RightPortType=output  PseudoPeriodic=off  Frequencies=[]  NoiseDistribution=none  NoiseParameters=[]  Unit=degC  AffineConversion=on  FilteringAndDerivatives=provide  SimscapeFilterOrder=1  InputFilterTimeConstant=0.001  UdotUserProvided=0
  Sum : Sum  Inputs=|+-
  Transfer Fcn : TransferFcn  Denominator=[3 1]
  Transfer Fcn1 : TransferFcn  Denominator=[1 1]
  CHUwi_mdot_kg/s_moisture : PMIOPort  Side=Right
  CHUwi_T_degC_moisture : PMIOPort  Port=2  Side=Right
  CHUwi_RH_%_moisture : PMIOPort  Port=3  Side=Right
  Outport : Outport
  Outport1 : Outport  Port=2
  moisture_extracted : Outport  Port=3
  wires:
  Transfer Fcn1/1 -> Simulink-PS Converter2/1
  T_Stack/1 -> Transfer Fcn1/1
  Transfer Fcn/1 -> Mux1/2, Simulink-PS Converter/1
  PS-Simulink Converter/1 -> Mux/2, Sum/2
  Mux1/1 -> Outport1/1
  Saturation/1 -> Mux1/1, Transfer Fcn/1
  Mux/1 -> Outport/1
  RH_set/1 -> Mux/1, Sum/1
  Sum/1 -> moisture_extracted/1, Saturation/1
  connections:
  Simulink-PS Converter/RConn1 -- CHUwi_T_degC_moisture/RConn1
  CHUwi_mdot_kg/s_moisture/RConn1 -- Simulink-PS Converter2/RConn1
  CHUwi_RH_%_moisture/RConn1 -- PS-Simulink Converter/LConn1

== system H175_Stage_01_Anode_Cathode/Controller/CWS-controller ==
  RH_set : Inport
  CWSo_RH_%_moisture : Inport  Port=2
  Mux : Mux  Inputs=2
  Mux1 : Mux  Inputs=2
  PID Controller : slpidlib/PID Controller  Controller=PI  Form=Parallel  TimeDomain=Continuous-time  UseExternalTs=off  SampleTime=-1  IntegratorMethod=Forward Euler  FilterMethod=Forward Euler  ControllerParametersSource=internal  P=1  I=1  UseKiTs=off  D=0  N=100  UseFilter=on  TunerSelectOption=Transfer Function Based (PID Tuner App)  InitialConditionSource=internal  InitialConditionForIntegrator=0  InitialConditionForFilter=0  DifferentiatorICPrevScaledInput=0  ExternalReset=none  TrackingMode=off  Kt=1  LimitOutput=on  SatLimitsSource=internal  UpperSaturationLimit=.2  LowerSaturationLimit=-.2  LinearizeAsGain=off  AntiWindupMode=none  Kb=1  LimitIntegrator=off  UpperIntegratorSaturationLimit=inf  LowerIntegratorSaturationLimit=-inf  POutMin=[]  POutMax=[]  IOutMin=[]  IOutMax=[]  DOutMin=[]  DOutMax=[]  NOutMin=[]  NOutMax=[]  SumOutMin=[]  SumOutMax=[]  SaturationOutMin=[]  SaturationOutMax=[]  PParamMin=[]  PParamMax=[]  IParamMin=[]  IParamMax=[]  DParamMin=[]  DParamMax=[]  NParamMin=[]  NParamMax=[]  KbParamMin=[]  KbParamMax=[]  KtParamMin=[]  KtParamMax=[]  KbOutMin=[]  KbOutMax=[]  KtOutMin=[]  KtOutMax=[]  IntegratorOutMin=[]  IntegratorOutMax=[]  FilterOutMin=[]  FilterOutMax=[]  SumI1OutMin=[]  SumI1OutMax=[]  SumI2OutMin=[]  SumI2OutMax=[]  SumI3OutMin=[]  SumI3OutMax=[]  SumI4OutMin=[]  SumI4OutMax=[]  SumDOutMin=[]  SumDOutMax=[]  DifferentiatorOutMin=[]  DifferentiatorOutMax=[]  FilterDiffOutCoefMin=[]  FilterDiffOutCoefMax=[]  ReciprocalOutMin=[]  ReciprocalOutMax=[]  SumDenOutMin=[]  SumDenOutMax=[]  SumNumOutMin=[]  SumNumOutMax=[]  DivideOutMin=[]  DivideOutMax=[]  UdiffTsProdOutMin=[]  UdiffTsProdOutMax=[]  NTsProdOutMin=[]  NTsProdOutMax=[]  UintegralTsProdOutMin=[]  UintegralTsProdOutMax=[]  UngainTsProdOutMin=[]  UngainTsProdOutMax=[]  ClampingZeroOutDataTypeStr=Inherit: Inherit via back propagation  ClampingZeroOutMin=[]  ClampingZeroOutMax=[]  FilterDenConstantOutDataTypeStr=Inherit: Inherit via back propagation  FilterDenConstantOutMin=[]  FilterDenConstantOutMax=[]  PCopyOutDataTypeStr=Inherit: Inherit via back propagation  PCopyOutMin=[]  PCopyOutMax=[]  NCopyOutDataTypeStr=Inherit: Inherit via back propagation  NCopyOutMin=[]  NCopyOutMax=[]  IntegratorContinuousStateAttributes=''  IntegratorStateMustResolveToSignalObject=off  IntegratorRTWStateStorageClass=Auto  FilterContinuousStateAttributes=''  FilterStateMustResolveToSignalObject=off  FilterRTWStateStorageClass=Auto  ParallelPVariant=InternalParameters  IdealPVariant=Disabled  IVariant=InternalParameters  DVariant=Disabled  IntegratorVariant=Continuous  SatVariant=Enabled  AWVariant=Passthrough  PCopyVariant=Disabled  TRVariant=Disabled  FdbkBlocksVariant=Forward  IdealPFdbkVariant=Disabled  SatFdbkVariant=Disabled  DerivativeFilterVariant=Disabled  NVariant=Disabled  NCopyVariant=Disabled_SignalSpec  FilterICVariant=Disabled  IntegratorICVariant=InternalICs  ExternalResetVariant=Disabled  TRSumVariant=Passthrough  SumFdbkVariant=Disabled  SumVariant=Sum_PI  TsampFilterVariant=InternalTs  TsampNgainVariant=Passthrough  TsampIntegralVariant=Disabled_SignalSpec  ExternalSaturationOutDataTypeStr=Inherit: Same as second input
  Simulink-PS Converter5 : nesl_utility/Simulink-PS Converter  PhysicalDomain=network_engine_domain  SubClassName=ps_input  LeftPortType=input  RightPortType=output  PseudoPeriodic=off  Frequencies=[]  NoiseDistribution=none  NoiseParameters=[]  Unit=kg/s  AffineConversion=off  FilteringAndDerivatives=provide  SimscapeFilterOrder=1  InputFilterTimeConstant=0.001  UdotUserProvided=0
  Sum : Sum  Inputs=|+-
  Transfer Fcn : TransferFcn  Denominator=[4 1]
  CWS_mdot_kg/s_moisture : PMIOPort  Side=Right
  Outport : Outport
  Outport1 : Outport  Port=2
  wires:
  Sum/1 -> PID Controller/1
  Transfer Fcn/1 -> Simulink-PS Converter5/1, Mux1/2
  CWSo_RH_%_moisture/1 -> Mux/2, Sum/2
  Mux1/1 -> Outport1/1
  PID Controller/1 -> Mux1/1, Transfer Fcn/1
  Mux/1 -> Outport/1
  RH_set/1 -> Mux/1, Sum/1
  connections:
  Simulink-PS Converter5/RConn1 -- CWS_mdot_kg/s_moisture/RConn1
